simulink model "untitled"  (R2012b)
settings: Solver=ode45  StartTime=0.0  StopTime=0.01  RelTol=1e-3
settings Model: Creator=André  LastModifiedBy=André

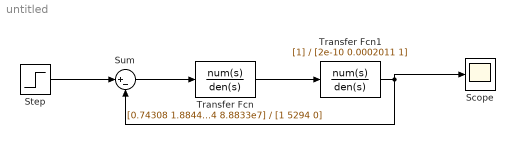
== system untitled ==
  Scope : Scope
      settings: TimeRange=1  YMin=-7  YMax=8
  Step : Step  Time=0  Before=1  SampleTime=0
  Sum : Sum  Inputs=|+-
  Transfer Fcn : TransferFcn  Numerator=[0.74308 1.8844e4 8.8833e7]  Denominator=[1 5294 0]
  Transfer Fcn1 : TransferFcn  Denominator=[2e-10 0.0002011 1]
  wires:
  Transfer Fcn/1 -> Transfer Fcn1/1
  Step/1 -> Sum/1
  Sum/1 -> Transfer Fcn/1
  Transfer Fcn1/1 -> Sum/2, Scope/1
